simulink model "emergency_scenario"  (R2023b)
settings: Solver=VariableStepAuto  StartTime=0.0  StopTime=1000  RelTol=1e-3
undefined symbols (not defined in the file or in its folder): entity, entitySys, get_Arrival, get_finalDeparture, m
settings Model: Creator=valet  LastModifiedBy=valet

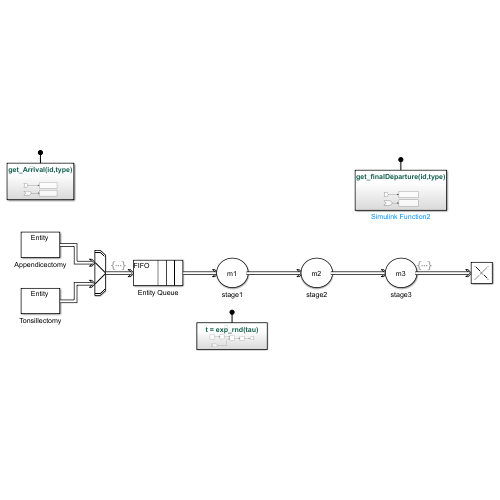
[thumbnail: Simulink's stored preview of the top-level diagram]
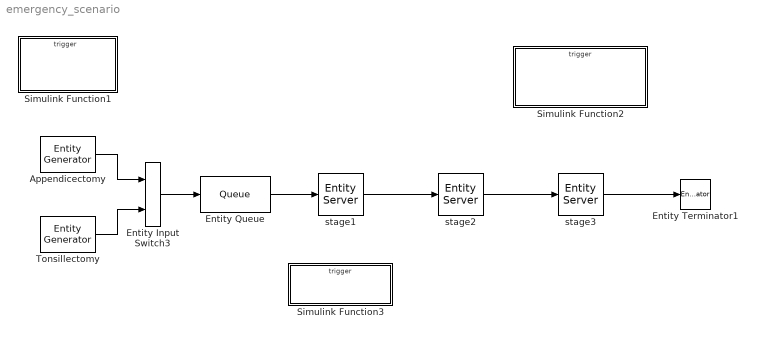
== system emergency_scenario ==
  Appendicectomy : EntityGenerator  OutputPortMessageModes=m  TimeSource=MATLAB action  IntergenerationTimeAction=dt = exp_rnd(1/lambdaA);  GenerateEntityAtSimulationStart=off  AttributeName=tau_1|tau_2|tau_3|type  AttributeInitialValue=tau_A_1|tau_A_2|tau_A_3|1  EntityType=Structured  EntityTypeName=Entity
  Entity Input Switch3 : EntityInputSwitch  InputPortMessageModes=m,m  OutputPortMessageModes=m
  Entity Queue : Queue  InputPortMessageModes=m  OutputPortMessageModes=m  Capacity=inf  EntryAction=get_Arrival(entitySys.id, entity.type)
  Entity Terminator1 : EntityTerminator  InputPortMessageModes=m
  Simulink Function1 : Subsystem  TreatAsAtomicUnit=on
  Simulink Function2 : Subsystem  TreatAsAtomicUnit=on
  Simulink Function3 : Subsystem  TreatAsAtomicUnit=on
  Tonsillectomy : EntityGenerator  OutputPortMessageModes=m  TimeSource=MATLAB action  IntergenerationTimeAction=dt = exp_rnd(1/lambdaT);  GenerateEntityAtSimulationStart=off  AttributeName=tau_1|tau_2|tau_3|type  AttributeInitialValue=tau_T_1|tau_T_2|tau_T_3|2  EntityType=Structured  EntityTypeName=Entity
  stage1 : EntityServer  InputPortMessageModes=m  OutputPortMessageModes=m  Capacity=m1  ServiceTimeSource=MATLAB action  ServiceTimeAction=dt = exp_rnd(entity.tau_1);
  stage2 : EntityServer  InputPortMessageModes=m  OutputPortMessageModes=m  Capacity=m2  ServiceTimeSource=MATLAB action  ServiceTimeAction=dt = exp_rnd(entity.tau_2);
  stage3 : EntityServer  InputPortMessageModes=m  OutputPortMessageModes=m  Capacity=m3  ServiceTimeSource=MATLAB action  ServiceTimeAction=dt = exp_rnd(entity.tau_3);  ExitAction=get_finalDeparture(entitySys.id, entity.type)
  wires:
  Tonsillectomy/1 -> Entity Input Switch3/2
  stage2/1 -> stage3/1
  Appendicectomy/1 -> Entity Input Switch3/1
  stage3/1 -> Entity Terminator1/1
  stage1/1 -> stage2/1
  Entity Queue/1 -> stage1/1
  Entity Input Switch3/1 -> Entity Queue/1

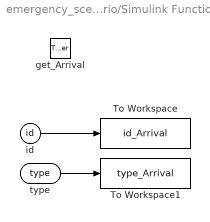
== system emergency_scenario/Simulink Function1 ==
  get_Arrival : TriggerPort  TriggerType=function-call  IsSimulinkFunction=on  FunctionName=get_Arrival  FunctionVisibility=scoped  VariantControl=(inherit)
  To Workspace : ToWorkspace  VariableName=id_Arrival  SaveFormat=Timeseries  SampleTime=-1
  To Workspace1 : ToWorkspace  VariableName=type_Arrival  SaveFormat=Timeseries  SampleTime=-1
  id : ArgIn  ArgumentName=id
  type : ArgIn  Port=2  ArgumentName=type
  wires:
  id/1 -> To Workspace/1
  type/1 -> To Workspace1/1

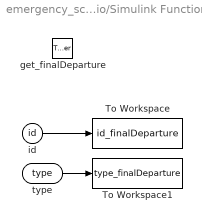
== system emergency_scenario/Simulink Function2 ==
  get_finalDeparture : TriggerPort  TriggerType=function-call  IsSimulinkFunction=on  FunctionName=get_finalDeparture  FunctionVisibility=scoped  VariantControl=(inherit)
  To Workspace : ToWorkspace  VariableName=id_finalDeparture  SaveFormat=Timeseries  SampleTime=-1
  To Workspace1 : ToWorkspace  VariableName=type_finalDeparture  SaveFormat=Timeseries  SampleTime=-1
  id : ArgIn  ArgumentName=id
  type : ArgIn  Port=2  ArgumentName=type
  wires:
  id/1 -> To Workspace/1
  type/1 -> To Workspace1/1

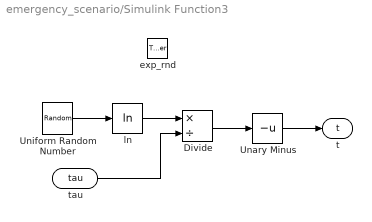
== system emergency_scenario/Simulink Function3 ==
  exp_rnd : TriggerPort  TriggerType=function-call  IsSimulinkFunction=on  FunctionName=exp_rnd  FunctionVisibility=scoped  VariantControl=(inherit)
  Divide : Product  Inputs=*/
  Unary Minus : UnaryMinus
  Uniform Random Number : UniformRandomNumber  Minimum=0
  ln : Math  Operator=log
  tau : ArgIn  ArgumentName=tau
  t : ArgOut  ArgumentName=t
  wires:
  Uniform Random Number/1 -> ln/1
  ln/1 -> Divide/1
  tau/1 -> Divide/2
  Divide/1 -> Unary Minus/1
  Unary Minus/1 -> t/1
